simulink model "task_3"  (R2024a)
settings: Solver=VariableStepAuto  StartTime=0.0  StopTime=100.0  RelTol=1e-3
settings Model: Creator=alexe  LastModifiedBy=alexe

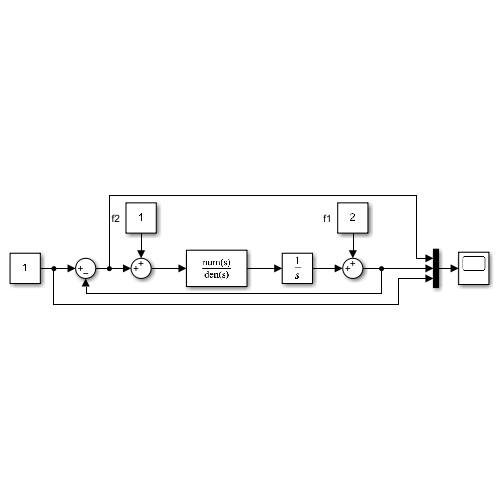
[thumbnail: Simulink's stored preview of the top-level diagram]
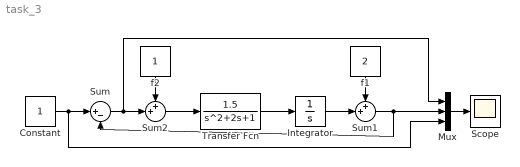
== system task_3 ==
  Constant : Constant
  Integrator : Integrator
  Mux : Mux  Inputs=3
  Scope : Scope
  Sum : Sum  Inputs=|+-
  Sum1 : Sum  Inputs=++|
  Sum2 : Sum  Inputs=++|
  Transfer Fcn : TransferFcn  Numerator=[1.5]
  f1 : Constant  Value=2
  f2 : Constant
  wires:
  Constant/1 -> Mux/3, Sum/1
  Sum/1 -> Mux/1, Sum2/2
  Sum2/1 -> Transfer Fcn/1
  Transfer Fcn/1 -> Integrator/1
  Integrator/1 -> Sum1/2
  Sum1/1 -> Sum/2, Mux/2
  Mux/1 -> Scope/1
  f2/1 -> Sum2/1
  f1/1 -> Sum1/1
